simulink model "contract1"  (R2015a)
settings: Solver=ode45  StartTime=0.0  StopTime=10.0  RelTol=1e-3
settings Model: Creator=teme  LastModifiedBy=teme

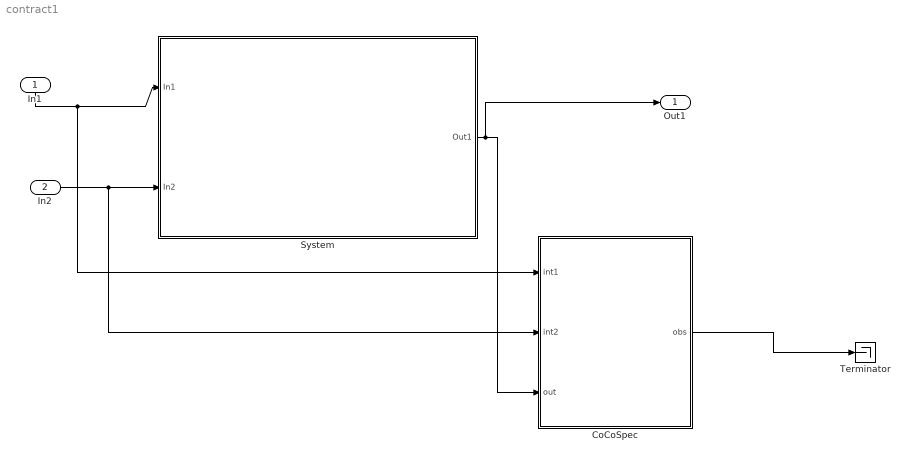
== system contract1 ==
  In1 : Inport  OutDataTypeStr=boolean
  In2 : Inport  Port=2  OutDataTypeStr=double
  CoCoSpec : MATLAB Function  TreatAsAtomicUnit=on
  System : Subsystem
  Terminator : Terminator
  Out1 : Outport
  wires:
  CoCoSpec/1(obs) -> Terminator/1
  In2/1 -> CoCoSpec/2(int2), System/2(In2)
  In1/1 -> CoCoSpec/1(int1), System/1(In1)
  System/1(Out1) -> Out1/1, CoCoSpec/3(out)

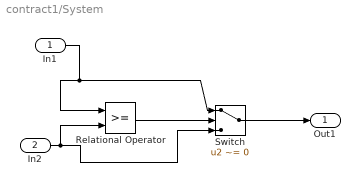
== system contract1/System ==
  In1 : Inport
  In2 : Inport  Port=2
  Relational Operator : RelationalOperator  OutDataTypeStr=boolean
  Switch : Switch  Criteria=u2 ~= 0
  Out1 : Outport
  wires:
  In1/1 -> Relational Operator/1, Switch/1
  In2/1 -> Relational Operator/2, Switch/3
  Relational Operator/1 -> Switch/2
  Switch/1 -> Out1/1

== matlab function contract1/CoCoSpec ==
  data: int1 input; obs output; int2 input; out input
function obs = fcn(int1, int2, out)

% cocospec (u) returns (y) 
% let
% --!assume
% tel

obs = true;
